simulink model "NavigationGUI"  (R2022b)
settings: Solver=VariableStepAuto  StartTime=0.0  StopTime=100  RelTol=1e-3
values from neighbouring files (symbols this model uses):
  floorl = 20    [EnvironmentData.mat]    (also in GUIWithNavigation.m; Practice data.mat; RunModel.m)
  floorw = 20    [EnvironmentData.mat]    (also in GUIWithNavigation.m; Practice data.mat; RunModel.m)
  startx = 3    [EnvironmentData.mat]    (also in Practice data.mat = 2)
  starty = 3    [EnvironmentData.mat]    (also in Practice data.mat = 2)
  target1 = [pthObj.States(:,1),pthObj.States(:,2)]    [GUIWithNavigation.m]    (also in RunModel.m)
  target2 = [pthObj.States(:,1),pthObj.States(:,2)]    [GUIWithNavigation.m]    (also in RunModel.m)
undefined symbols (not defined in the file or in its folder): X, Y, Z
libraries: sm_lib x66, nesl_utility x10, slpidlib x3
(part 2 of 2)

== matlab function NavigationGUI/Sensors/MATLAB Function ==
  settings: updateMethod=DISCRETE
  data: forwardVelocity output; angVelocity output; target1 input; target2 input; xpos input; ypos input; anglePos input; stopSim output; debug output
function [forwardVelocity,angVelocity,stopSim,debug] = pathChaser(target1,target2,xpos,ypos,anglePos)


%used to keep track of the current target
persistent currentTarget;
persistent path;

if isempty(currentTarget)
    currentTarget = 1;
end

if isempty(path)
    path =1;
end





rotMoveSpeed=1;
if path==1
    target=target1;
elseif path==2
    target=target2;
else
    target=target1;
end

%finds the number of targets
numTargets=size(target,1);
%sets the variable that stops the simulation to 0
stopSim=0;
%gets the x and y positions of the current target
targetx=target(currentTarget,1);
targety=target(currentTarget,2);

%finds the distance between the body of the robot and the target centre
xDiff=targetx-xpos;
yDiff=targety-ypos;
%finds the angle between the x axis of the simulation and the line pointing
%towards the target centre
targetAngle=atan2(yDiff,xDiff);

%finds the angle between the x axis of the robot and the line pointing
%toward the target centre
angDiff=targetAngle-anglePos;

%checkis if the robot has reached the final target
if currentTarget==numTargets
    if path==1
        forwardVelocity=0;
        angVelocity=0;
        pause(5);
        currentTarget=1;
        path=2;
    elseif path==2
        stopSim=1;
        forwardVelocity=0;
        angVelocity=0;
    else
       forwardVelocity=0;
        angVelocity=0; 
    end

%if not runs the path follower
else 
    %if the robot is not within 0.1m of the target
    if abs(xDiff+yDiff)>=0.1
        %if the angle between the x axis of the robot and the target is not
        %less than ~6 degrees
        if abs(angDiff)>=0.05
            %if the angle difference is positive
            if angDiff>0
                %stop and rotate left
                angVelocity=rotMoveSpeed;
                forwardVelocity=0;
            else
                %else stop and rotate right
                angVelocity=-rotMoveSpeed;
                forwardVelocity=0;
            end
        else
            %if angle is less than ~6 degrees move forward
            angVelocity=0;
            forwardVelocity=1;
        end

    else
        %if robot is within 0.1m of target check target off and set new
        %target
        currentTarget=currentTarget+1;
        forwardVelocity=0;
        angVelocity=0;
    end
end
debug=currentTarget;
